simulink model "ass6_6"  (R2023a)
settings: Solver=VariableStepAuto  StartTime=0.0  StopTime=10.0  RelTol=1e-3
settings Model: Creator=Taniya Baral  LastModifiedBy=Taniya Baral

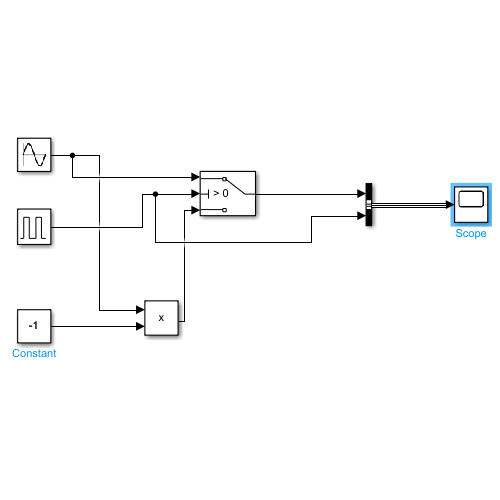
[thumbnail: Simulink's stored preview of the top-level diagram]
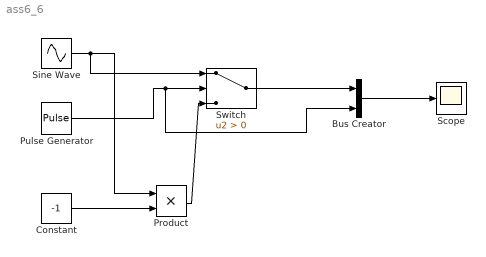
== system ass6_6 ==
  Bus Creator : BusCreator  Inputs=2
  Constant : Constant  Value=-1
  Product : Product
  Pulse Generator : DiscretePulseGenerator  PulseType=Time based  Period=20  PulseWidth=5
  Scope : Scope
  Sine Wave : Sin  Frequency=2*pi  Phase=180  SampleTime=0
  Switch : Switch  Criteria=u2 > Threshold  SaturateOnIntegerOverflow=off  InputSameDT=off
  wires:
  Sine Wave/1 -> Switch/1, Product/1
  Constant/1 -> Product/2
  Product/1 -> Switch/3
  Pulse Generator/1 -> Bus Creator/2, Switch/2
  Switch/1 -> Bus Creator/1
  Bus Creator/1 -> Scope/1
